simulink model "CAES_Expansion"  (R2022a)
settings: Solver=VariableStepAuto  StartTime=0.0  StopTime=100  RelTol=1e-3
values from neighbouring files (symbols this model uses):
  c1 = 1-c2    (= 0.95)    [CAES_Parameters.m]
  c2 = 0.05    [CAES_Parameters.m]
  Dt = 2    [CAES_Parameters.m]
  Fmax = 1.25+0.25    (= 1.5)    [CAES_Parameters.m]
  Fmin = 0    [CAES_Parameters.m]
  gmax = 1.25+0.25    (= 1.5)    [CAES_Parameters.m]
  gmin = 0.1    [CAES_Parameters.m]
  Ht = 3.9821    [CAES_Parameters.m]
  K4 = 0.8    [CAES_Parameters.m]
  K5 = 0.2    [CAES_Parameters.m]
  Kti = 2    [CAES_Parameters.m]
  KTi = 5    [CAES_Parameters.m]
  Ktp = 3    [CAES_Parameters.m]
  KTp = 7    [CAES_Parameters.m]
  R = 0.04    [CAES_Parameters.m]
  tau3 = 15    [CAES_Parameters.m]
  tau4 = 2.5    [CAES_Parameters.m]
  tauAV = 0.1    [CAES_Parameters.m]
  tauS = 0.05    [CAES_Parameters.m]
  tauSF = 0.4    [CAES_Parameters.m]
  tauTD = 0.3    [CAES_Parameters.m]
  tauTP = 0.02    [CAES_Parameters.m]
  Ts = 323.15    [CAES_Parameters.m]
  TxLPo = 668.15    [CAES_Parameters.m]
  Txref = 1    [CAES_Parameters.m]
  umax = 1.2+0.3    (= 1.5)    [CAES_Parameters.m]
  umin = 0    [CAES_Parameters.m]
libraries: slpidlib x2, spsGroundLib x2, spsLoadFlowBusLib x2, spsThreePhaseParallelRLCLoadLib x2, spsThreePhaseBreakerLib x1, spsSimplifiedSynchronousMachinepuUnitsLib x1, spspowerguiLib x1, spsVoltageMeasurementLib x1
settings Model: Creator=xiaojs20  LastModifiedBy=xiaojs20

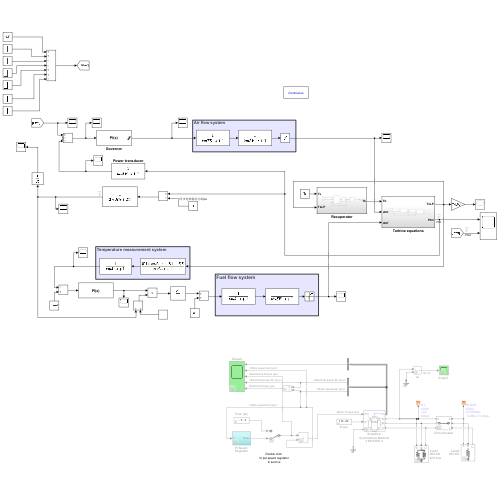
[thumbnail: Simulink's stored preview of the top-level diagram]
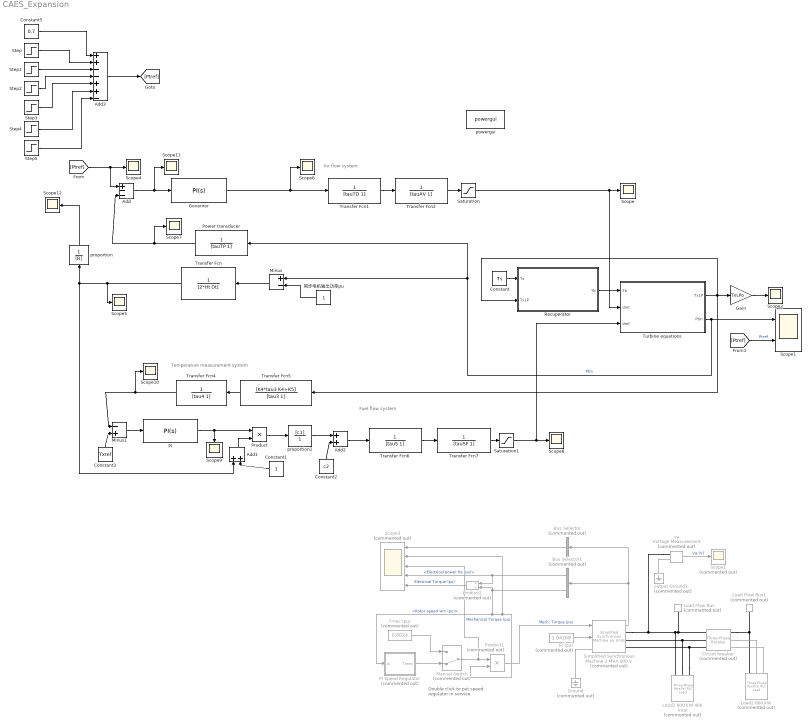
== system CAES_Expansion ==
  note: Fuel flow system
  note: Temperature measurement system
  note: Air flow system
  note: Double click
      | to put speed regulator
      | in service
  Add : Sum  Inputs=+--
  Add1 : Sum
  Add2 : Sum
  Add3 : Sum  Inputs=++--++-
  Bus Selector : BusSelector  Commented=on  OutputSignals=Stator current is_a (pu),Stator current is_b (pu),Stator current is_c (pu)  OutputAsBus=on
  Bus Selector1 : BusSelector  Commented=on  OutputSignals=Electrical power Pe (pu),Rotor speed wm (pu)
  Circuit breaker : spsThreePhaseBreakerLib/Three-Phase Breaker  Commented=on  InitialState=closed  SwitchA=on  SwitchB=on  SwitchC=on  SwitchTimes=[ 0.2 0.7*100 ]  External=off  BreakerResistance=1e-4  SnubberResistance=inf  SnubberCapacitance=0  Measurements=None
      settings: AttributesFormatString=\n
  Constant : Constant  Value=Ts
  Constant1 : Constant
  Constant2 : Constant  Value=c2
  Constant3 : Constant  Value=Txref
  Constant5 : Constant  Value=0.7
  Ei (pu) : Constant  Commented=on  Value=1.04268
  Gain : Gain  Gain=TxLPo
  Governor : slpidlib/PID Controller  Controller=PI  Form=Parallel  TimeDomain=Continuous-time  UseExternalTs=off  SampleTime=-1  IntegratorMethod=Forward Euler  FilterMethod=Forward Euler  ControllerParametersSource=internal  P=Ktp  I=Kti  UseKiTs=off  D=0  N=100  UseFilter=on  TunerSelectOption=Transfer Function Based (PID Tuner App)  InitialConditionSource=internal  InitialConditionForIntegrator=0  InitialConditionForFilter=0  DifferentiatorICPrevScaledInput=0  ExternalReset=none  TrackingMode=off  Kt=1  LimitOutput=on  SatLimitsSource=internal  UpperSaturationLimit=umax  LowerSaturationLimit=umin  LinearizeAsGain=on  AntiWindupMode=none  Kb=1  POutMin=[]  POutMax=[]  IOutMin=[]  IOutMax=[]  DOutMin=[]  DOutMax=[]  NOutMin=[]  NOutMax=[]  SumOutMin=[]  SumOutMax=[]  SaturationOutMin=[]  SaturationOutMax=[]  PParamMin=[]  PParamMax=[]  IParamMin=[]  IParamMax=[]  DParamMin=[]  DParamMax=[]  NParamMin=[]  NParamMax=[]  KbParamMin=[]  KbParamMax=[]  KtParamMin=[]  KtParamMax=[]  KbOutMin=[]  KbOutMax=[]  KtOutMin=[]  KtOutMax=[]  IntegratorOutMin=[]  IntegratorOutMax=[]  FilterOutMin=[]  FilterOutMax=[]  SumI1OutMin=[]  SumI1OutMax=[]  SumI2OutMin=[]  SumI2OutMax=[]  SumI3OutMin=[]  SumI3OutMax=[]  SumI4OutMin=[]  SumI4OutMax=[]  SumDOutMin=[]  SumDOutMax=[]  DifferentiatorOutMin=[]  DifferentiatorOutMax=[]  FilterDiffOutCoefMin=[]  FilterDiffOutCoefMax=[]  ReciprocalOutMin=[]  ReciprocalOutMax=[]  SumDenOutMin=[]  SumDenOutMax=[]  SumNumOutMin=[]  SumNumOutMax=[]  DivideOutMin=[]  DivideOutMax=[]  UdiffTsProdOutMin=[]  UdiffTsProdOutMax=[]  NTsProdOutMin=[]  NTsProdOutMax=[]  UintegralTsProdOutMin=[]  UintegralTsProdOutMax=[]  UngainTsProdOutMin=[]  UngainTsProdOutMax=[]  IntegratorContinuousStateAttributes=''  IntegratorStateMustResolveToSignalObject=off  IntegratorRTWStateStorageClass=Auto  FilterContinuousStateAttributes=''  FilterStateMustResolveToSignalObject=off  FilterRTWStateStorageClass=Auto  ParallelPVariant=InternalParameters  IdealPVariant=Disabled  IVariant=InternalParameters  DVariant=Disabled  IntegratorVariant=Continuous  SatVariant=Enabled  AWVariant=Passthrough  PCopyVariant=Disabled  TRVariant=Disabled  FdbkBlocksVariant=Forward  IdealPFdbkVariant=Disabled  SatFdbkVariant=Disabled  DerivativeFilterVariant=Disabled  NVariant=Disabled  NCopyVariant=Disabled_SignalSpec  FilterICVariant=Disabled  IntegratorICVariant=InternalICs  ExternalResetVariant=Disabled  TRSumVariant=Passthrough  SumFdbkVariant=Disabled  SumVariant=Sum_PI  TsampFilterVariant=InternalTs  TsampNgainVariant=Passthrough  TsampIntegralVariant=Passthrough  ExternalSaturationOutDataTypeStr=Inherit: Same as second input  aMode=0
  Ground : spsGroundLib/Ground  Commented=on  LConnTagsString=a
  Load Flow Bus : spsLoadFlowBusLib/Load Flow Bus  Commented=on  LConnTagsString=a  Phases=single  Connectors=on one side  ID=B1  Vbase=600  Vref=1  Vangle=0  VLF=1  VLFb=1  VLFc=1  angleLF=0  angleLFb=0  angleLFc=0
      settings: AttributesFormatString=%<ID>\n%<Vbase>V\n%<VLF>pu\n%<angleLF>deg.  SourceProductBaseCode=PS
  Load Flow Bus1 : spsLoadFlowBusLib/Load Flow Bus  Commented=on  LConnTagsString=a  Phases=single  Connectors=on one side  ID=BLOAD  Vbase=600  Vref=1  Vangle=0  VLF=0.9998  VLFb=1  VLFc=1  angleLF=-9.68e-011  angleLFb=0  angleLFc=0
      settings: AttributesFormatString=%<ID>\n%<Vbase>V\n%<VLF>pu\n%<angleLF>deg.  SourceProductBaseCode=PS
  Load1 800 kW 400 kvar : spsThreePhaseParallelRLCLoadLib/Three-Phase Parallel RLC Load  Commented=on  LConnTagsString=A|B|C  Configuration=Y (grounded)  NominalVoltage=600  Vabc=[1e3 1e3 1e3]  Vabcp=[1e3 1e3 1e3]  NominalFrequency=60  UnbalancedPower=off  ActivePower=800000  InductivePower=400e3  CapacitivePower=0  Pabc=[10e3 9e3 11e3]  QLabc=[100 90 110]  QCabc=[100 90 110]  Pabcp=[10e3 9e3 11e3]  QLabcp=[100 90 110]  QCabcp=[100 90 110]  Measurements=None  LoadType=constant Z
  Load2 800 kW : spsThreePhaseParallelRLCLoadLib/Three-Phase Parallel RLC Load  Commented=on  LConnTagsString=A|B|C  Configuration=Y (grounded)  NominalVoltage=600  Vabc=[1e3 1e3 1e3]  Vabcp=[1e3 1e3 1e3]  NominalFrequency=60  UnbalancedPower=off  ActivePower=800000  InductivePower=0  CapacitivePower=0  Pabc=[10e3 9e3 11e3]  QLabc=[100 90 110]  QCabc=[100 90 110]  Pabcp=[10e3 9e3 11e3]  QLabcp=[100 90 110]  QCabcp=[100 90 110]  Measurements=None  LoadType=constant Z
  Manual Switch : ManualSwitch  Commented=on  CurrentSetting=0
  Minus : Sum  Inputs=+-
  Minus1 : Sum  Inputs=-+
  PI : slpidlib/PID Controller  Controller=PI  Form=Parallel  TimeDomain=Continuous-time  UseExternalTs=off  SampleTime=-1  IntegratorMethod=Forward Euler  FilterMethod=Forward Euler  ControllerParametersSource=internal  P=KTp  I=KTi  UseKiTs=off  D=0  N=100  UseFilter=on  TunerSelectOption=Transfer Function Based (PID Tuner App)  InitialConditionSource=internal  InitialConditionForIntegrator=0  InitialConditionForFilter=0  DifferentiatorICPrevScaledInput=0  ExternalReset=none  TrackingMode=off  Kt=1  LimitOutput=off  SatLimitsSource=internal  UpperSaturationLimit=umax  LowerSaturationLimit=umin  LinearizeAsGain=on  AntiWindupMode=none  Kb=1  POutMin=[]  POutMax=[]  IOutMin=[]  IOutMax=[]  DOutMin=[]  DOutMax=[]  NOutMin=[]  NOutMax=[]  SumOutMin=[]  SumOutMax=[]  SaturationOutMin=[]  SaturationOutMax=[]  PParamMin=[]  PParamMax=[]  IParamMin=[]  IParamMax=[]  DParamMin=[]  DParamMax=[]  NParamMin=[]  NParamMax=[]  KbParamMin=[]  KbParamMax=[]  KtParamMin=[]  KtParamMax=[]  KbOutMin=[]  KbOutMax=[]  KtOutMin=[]  KtOutMax=[]  IntegratorOutMin=[]  IntegratorOutMax=[]  FilterOutMin=[]  FilterOutMax=[]  SumI1OutMin=[]  SumI1OutMax=[]  SumI2OutMin=[]  SumI2OutMax=[]  SumI3OutMin=[]  SumI3OutMax=[]  SumI4OutMin=[]  SumI4OutMax=[]  SumDOutMin=[]  SumDOutMax=[]  DifferentiatorOutMin=[]  DifferentiatorOutMax=[]  FilterDiffOutCoefMin=[]  FilterDiffOutCoefMax=[]  ReciprocalOutMin=[]  ReciprocalOutMax=[]  SumDenOutMin=[]  SumDenOutMax=[]  SumNumOutMin=[]  SumNumOutMax=[]  DivideOutMin=[]  DivideOutMax=[]  UdiffTsProdOutMin=[]  UdiffTsProdOutMax=[]  NTsProdOutMin=[]  NTsProdOutMax=[]  UintegralTsProdOutMin=[]  UintegralTsProdOutMax=[]  UngainTsProdOutMin=[]  UngainTsProdOutMax=[]  IntegratorContinuousStateAttributes=''  IntegratorStateMustResolveToSignalObject=off  IntegratorRTWStateStorageClass=Auto  FilterContinuousStateAttributes=''  FilterStateMustResolveToSignalObject=off  FilterRTWStateStorageClass=Auto  ParallelPVariant=InternalParameters  IdealPVariant=Disabled  IVariant=InternalParameters  DVariant=Disabled  IntegratorVariant=Continuous  SatVariant=Disabled  AWVariant=Passthrough  PCopyVariant=Disabled  TRVariant=Disabled  FdbkBlocksVariant=Forward  IdealPFdbkVariant=Disabled  SatFdbkVariant=Disabled  DerivativeFilterVariant=Disabled  NVariant=Disabled  NCopyVariant=Disabled_SignalSpec  FilterICVariant=Disabled  IntegratorICVariant=InternalICs  ExternalResetVariant=Disabled  TRSumVariant=Passthrough  SumFdbkVariant=Disabled  SumVariant=Sum_PI  TsampFilterVariant=InternalTs  TsampNgainVariant=Passthrough  TsampIntegralVariant=Passthrough  ExternalSaturationOutDataTypeStr=Inherit: Same as second input  aMode=0
  PI Speed Regulator : Subsystem  Commented=on
  Power transducer : TransferFcn  Denominator=[tauTP 1]
  Product : Product
  Product1 : Product  Commented=on  InputSameDT=on  SaturateOnIntegerOverflow=on  OutDataTypeStr=Inherit: Same as first input
  Product2 : Product  Commented=on  Inputs=*/  InputSameDT=on  SaturateOnIntegerOverflow=on  OutDataTypeStr=Inherit: Same as first input
  Recuperator : Subsystem
  Saturation : Saturate  UpperLimit=gmax  LowerLimit=gmin
  Saturation1 : Saturate  UpperLimit=Fmax  LowerLimit=Fmin  ZeroCross=off
  Scope{,2,4..12} (11 alike) : Scope
  Scope1 : Scope  NumInputPorts=2
  "Scope1 " : Scope  Commented=on
  Scope3 : Scope  Commented=on  NumInputPorts=5
  Simplified Synchronous Machine 2 MVA 600 V : spsSimplifiedSynchronousMachinepuUnitsLib/Simplified Synchronous Machine pu Units  Commented=on  ConnectionType=4-wire Y  MechanicalLoad=Mechanical power Pm  MeasurementBus=off  NominalParameters="[  2000e3, 600, 60 ]"  Mechanical=[ 0.6 , 0.0, 2 ]  InternalRL="[ 0.0036  0.16 ]"  InitialConditions=[0 7.01083 0.824535 0.824535 0.824535 -14.0377 -134.038 105.962 ]  IterativeDiscreteModel=Trapezoidal non iterative  TsBlock=-1  TsPowergui=0  LoadFlowParameters=[2 0 0 0]  Units=0  BusType=swing  Pref=0  Qref=0  Qmin=-Inf  Qmax=Inf  PLF=0  QLF=0
      settings: AttributesFormatString=\n  SourceProductBaseCode=PS
  Step : Step  Time=5  After=0.3  SampleTime=0  ZeroCross=off
  Step1 : Step  Time=20  After=0.3  SampleTime=0  ZeroCross=off
  Step2 : Step  Time=35  After=0.1  SampleTime=0  ZeroCross=off
  Step3 : Step  Time=50  After=0.1  SampleTime=0  ZeroCross=off
  Step4 : Step  Time=65  After=0.5  SampleTime=0  ZeroCross=off
  Step5 : Step  Time=80  After=0.5  SampleTime=0  ZeroCross=off
  Tmec (pu) : Constant  Commented=on  Value=0.8024
  Transfer Fcn : TransferFcn  Denominator=[2*Ht Dt]
  Transfer Fcn1 : TransferFcn  Denominator=[tauTD 1]
  Transfer Fcn2 : TransferFcn  Denominator=[tauAV 1]
  Transfer Fcn4 : TransferFcn  Denominator=[tau4 1]
  Transfer Fcn5 : TransferFcn  Numerator=[K4*tau3 K4+K5]  Denominator=[tau3 1]
  Transfer Fcn6 : TransferFcn  Denominator=[tauS 1]
  Transfer Fcn7 : TransferFcn  Denominator=[tauSF 1]
  Turbine equations : Subsystem
  output Ground1 : spsGroundLib/Ground  Commented=on  LConnTagsString=a
  powergui : spspowerguiLib/powergui  Priority=1  SimulationMode=Continuous  SampleTime=50e-6  frequency=60  Iterations=50  frequencyindice=60  Pbase=100e6  ErrMax=1e-4  UnitsV=kV  UnitsW=MW  buscounter=0  FunctionMessages=off  echomessages=off  EnableUseOfTLC=off  CurrentSourceSwitches=off  DisableSnubberDevices=off  DisableRonSwitches=off  DisableVfSwitches=off  DisplayEquations=off  AutomaticDiscreteSolvers=off  SolverType=Tustin/Backward Euler (TBE)  Interpol=off  ExternalGateDelay=off  methode=off  Ts=100  x0status=blocks  SPID=on  SwTol=0  HookPort=off  NonlinearTolerance=1e-4  nMaxIteration=100  ContinueOnMaxIteration=off  RestoreLinks=warning  ResistiveCurrentMeasurement=off  Frange=[0:2:500]  Ylog=off  Xlog=on  ShowGrid=off  save=off  variable=ZData  structure=0  ZoomFFT=off  StartTime=0.0  cycles=1  DisplayStyle=1  fundamental=60  FreqAxis=off  MaxFrequency=1000  frequencyindicesteady=1  RmsSteady=1  display=off
  proportion : TransferFcn  Denominator=[R]
  proportion1 : TransferFcn  Numerator=[c1]  Denominator=[1]
  va : spsVoltageMeasurementLib/Voltage Measurement  Tag=PoWeRsYsTeMmEaSuReMeNt  Commented=on  PhasorSimulation=off  OutputType=Magnitude  PSBequivalent=0
  同步电机输出功率pu : Constant
  wires:
  Transfer Fcn/1 -> Scope5/1, Add1/1, proportion/1
  Minus/1 -> Transfer Fcn/1
  Turbine equations/2(Ptm) -> Power transducer/1, Minus/1, Scope1/1  "Ptm"
  Governor/1 -> Scope6/1, Transfer Fcn1/1
  Transfer Fcn1/1 -> Transfer Fcn2/1
  Transfer Fcn2/1 -> Saturation/1
  Add/1 -> Scope11/1, Governor/1
  Power transducer/1 -> Scope7/1, Add/3
  Turbine equations/1(TxLP) -> Gain/1, Transfer Fcn5/1, Recuperator/2(TxLP)
  Transfer Fcn5/1 -> Transfer Fcn4/1
  Transfer Fcn4/1 -> Scope10/1, Minus1/1
  Minus1/1 -> PI/1
  Constant3/1 -> Minus1/2
  PI/1 -> Product/1, Scope9/1
  Constant1/1 -> Add1/2
  Add1/1 -> Product/2
  Product/1 -> proportion1/1
  proportion1/1 -> Add2/1
  Constant2/1 -> Add2/2
  Add2/1 -> Transfer Fcn6/1
  Transfer Fcn6/1 -> Transfer Fcn7/1
  Transfer Fcn7/1 -> Saturation1/1
  Recuperator/1(Tb) -> Turbine equations/1(Tb)
  Saturation/1 -> Scope/1, Turbine equations/2(dmt)
  Saturation1/1 -> Scope8/1, Turbine equations/3(dmf)
  Constant/1 -> Recuperator/1(Ts)
  Add3/1 -> [Ptref]
  Step/1 -> Add3/2
  Constant5/1 -> Add3/1
  Step1/1 -> Add3/3
  Step2/1 -> Add3/4
  Step3/1 -> Add3/5
  Step4/1 -> Add3/6
  Step5/1 -> Add3/7
  [Ptref] -> Add/1, Scope4/1
  Bus Selector1/1 -> Product2/1, Scope3/4  "<Electrical power Pe (pu)>"
  Simplified Synchronous Machine 2 MVA 600 V/1 -> Bus Selector1/1, Bus Selector/1
  Bus Selector1/2 -> PI Speed Regulator/1(w), Scope3/2, Product1/2, Product2/2  "<Rotor speed wm (pu)>"
  Product1/1 -> Simplified Synchronous Machine 2 MVA 600 V/1  "Mech. Torque (pu)"
  Bus Selector/1 -> Scope3/1
  Product2/1 -> Scope3/5  "Electrical Torque (pu)"
  Manual Switch/1 -> Product1/1, Scope3/3  "Mechanical Torque (pu)"
  Ei (pu)/1 -> Simplified Synchronous Machine 2 MVA 600 V/2
  va/1 -> "Scope1 "/1  "Va (V)"
  PI Speed Regulator/1(Tmec) -> Manual Switch/2
  Tmec (pu)/1 -> Manual Switch/1
  [Ptref] -> Scope1/2  "Ptref"
  proportion/1 -> Scope12/1
  Gain/1 -> Scope2/1
  同步电机输出功率pu/1 -> Minus/2
  connections:
  va/LConn1 -- Circuit breaker/LConn1 -- Load Flow Bus/LConn1 -- Load1 800 kW 400 kvar/LConn1 -- Simplified Synchronous Machine 2 MVA 600 V/RConn1
  Load1 800 kW 400 kvar/LConn2 -- Circuit breaker/LConn2 -- Simplified Synchronous Machine 2 MVA 600 V/RConn2
  Load Flow Bus1/LConn1 -- Circuit breaker/RConn1 -- Load2 800 kW/LConn1
  Load1 800 kW 400 kvar/LConn3 -- Circuit breaker/LConn3 -- Simplified Synchronous Machine 2 MVA 600 V/RConn3
  output Ground1/LConn1 -- va/LConn2
  Simplified Synchronous Machine 2 MVA 600 V/LConn1 -- Ground/LConn1
  Circuit breaker/RConn2 -- Load2 800 kW/LConn2
  Circuit breaker/RConn3 -- Load2 800 kW/LConn3

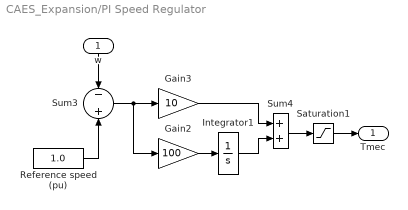
== system CAES_Expansion/PI Speed Regulator ==
  w : Inport
  Gain2 : Gain  Gain=100  SaturateOnIntegerOverflow=on  OutDataTypeStr=Inherit: Same as input  ParamDataTypeStr=Inherit: Same as input
  Gain3 : Gain  Gain=10  SaturateOnIntegerOverflow=on  OutDataTypeStr=Inherit: Same as input  ParamDataTypeStr=Inherit: Same as input
  Integrator1 : Integrator  InitialCondition=0.8024  LimitOutput=on  UpperSaturationLimit=1  LowerSaturationLimit=0  ZeroCross=off
  Reference speed (pu) : Constant  Value=1.0
  Saturation1 : Saturate  UpperLimit=1  LowerLimit=0  ZeroCross=off
  Sum3 : Sum  Inputs=-+  InputSameDT=on  SaturateOnIntegerOverflow=on  OutDataTypeStr=Inherit: Same as first input
  Sum4 : Sum  InputSameDT=on  SaturateOnIntegerOverflow=on  OutDataTypeStr=Inherit: Same as first input
  Tmec : Outport  VectorParamsAs1DForOutWhenUnconnected=off
  wires:
  Gain3/1 -> Sum4/1
  Gain2/1 -> Integrator1/1
  Sum3/1 -> Gain3/1, Gain2/1
  Integrator1/1 -> Sum4/2
  Reference speed (pu)/1 -> Sum3/2
  Sum4/1 -> Saturation1/1
  w/1 -> Sum3/1
  Saturation1/1 -> Tmec/1

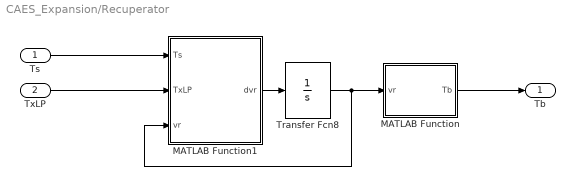
== system CAES_Expansion/Recuperator ==
  Ts : Inport
  TxLP : Inport  Port=2
  MATLAB Function : MATLAB Function  TreatAsAtomicUnit=on
  MATLAB Function1 : MATLAB Function  TreatAsAtomicUnit=on
  Transfer Fcn8 : TransferFcn  Denominator=[1 0]
  Tb : Outport
  wires:
  MATLAB Function1/1(dvr) -> Transfer Fcn8/1
  TxLP/1 -> MATLAB Function1/2(TxLP)
  Transfer Fcn8/1 -> MATLAB Function/1(vr), MATLAB Function1/3(vr)
  MATLAB Function/1(Tb) -> Tb/1
  Ts/1 -> MATLAB Function1/1(Ts)

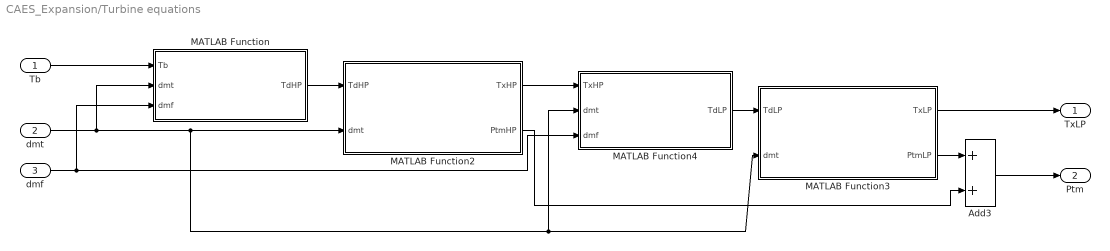
== system CAES_Expansion/Turbine equations ==
  Tb : Inport
  dmt : Inport  Port=2
  dmf : Inport  Port=3
  Add3 : Sum
  MATLAB Function : MATLAB Function  TreatAsAtomicUnit=on
  MATLAB Function2 : MATLAB Function  TreatAsAtomicUnit=on
  MATLAB Function3 : MATLAB Function  TreatAsAtomicUnit=on
  MATLAB Function4 : MATLAB Function  TreatAsAtomicUnit=on
  TxLP : Outport
  Ptm : Outport  Port=2
  wires:
  MATLAB Function2/2(PtmHP) -> Add3/2
  Add3/1 -> Ptm/1
  dmf/1 -> MATLAB Function4/3(dmf), MATLAB Function/3(dmf)
  dmt/1 -> MATLAB Function/2(dmt), MATLAB Function4/2(dmt), MATLAB Function3/2(dmt), MATLAB Function2/2(dmt)
  MATLAB Function/1(TdHP) -> MATLAB Function2/1(TdHP)
  Tb/1 -> MATLAB Function/1(Tb)
  MATLAB Function3/2(PtmLP) -> Add3/1
  MATLAB Function3/1(TxLP) -> TxLP/1
  MATLAB Function4/1(TdLP) -> MATLAB Function3/1(TdLP)
  MATLAB Function2/1(TxHP) -> MATLAB Function4/1(TxHP)

== matlab function CAES_Expansion/Recuperator/MATLAB Function1 ==
  data: dvr output; Ts input; TxLP input; vr input
function dvr=dvr_solver(Ts,TxLP,vr)
    TxLPo=668.15;
    Tbo=599.15;
    eps_r=0.80;
    tauR=25;

    dvr=(1/tauR)*(eps_r*(TxLP*TxLPo-Ts)/(Tbo)-vr);
end

== matlab function CAES_Expansion/Recuperator/MATLAB Function ==
  data: Tb output; vr input
function Tb=Tb_solver(vr)
    Ts=323.15;
    Tbo=599.15;
    Tb=Ts/Tbo+vr;
end

== matlab function CAES_Expansion/Turbine equations/MATLAB Function ==
  data: Tb input; TdHP output; dmt input; dmf input
function TdHP=HPburner_solver(Tb,dmt,dmf)
    Tbo=599.15;
    TdHPo=823.15; 

    TdHP=Tb*(Tbo/TdHPo)+((TdHPo-Tbo)/TdHPo)*(dmf/dmt);
end

== matlab function CAES_Expansion/Turbine equations/MATLAB Function2 ==
  data: TdHP input; dmt input; TxHP output; PtmHP output
function [TxHP,PtmHP]=HPexpander_solver(TdHP,dmt)
    TdHPo=823.15; 
    TxHPo=612.15;
    gamma=1.4;
    g=(gamma-1)/gamma;
    pi_tHPo=3.818;
    eta_tHPi=0.8065;
    cp=1.055;
    Ptmo=280;
    dmto=417;

    TxHP=(TdHPo*TdHP)/TxHPo*(1-(1-1/(pi_tHPo*dmt)^g)*eta_tHPi);
    PtmHP=(eta_tHPi*cp*dmto)/(1e3*Ptmo)*dmt*(TdHPo*TdHP-TxHPo*TxHP);

end

== matlab function CAES_Expansion/Turbine equations/MATLAB Function3 ==
  data: TdLP input; dmt input; TxLP output; PtmLP output
function [TxLP,PtmLP]=LPexpander_solver(TdLP,dmt)
    TdHPo=823.15; TdLPo=1098.2; TxHPo=612.15; TxLPo=668.15;
    gamma=1.4;
    g=(gamma-1)/gamma;
    pi_tHPo=3.818; pi_tLPo=10.856;
    eta_tHPi=0.8065; eta_tLPi=0.7926;
    cp=1.055;
    Ptmo=280;
    dmto=417;

    TxLP=(TdLPo*TdLP)/TxLPo*(1-(1-1/(pi_tLPo*dmt)^g)*eta_tLPi);
    PtmLP=(eta_tLPi*cp*dmto)/(1e3*Ptmo)*dmt*(TdLPo*TdLP-TxLPo*TxLP);

end

== matlab function CAES_Expansion/Turbine equations/MATLAB Function4 ==
  data: TxHP input; TdLP output; dmt input; dmf input
function TdLP=LPburner_solver(TxHP,dmt,dmf)
    Tbo=599.15;
    TdHPo=823.15; TdLPo=1098.2; TxHPo=612.15; TxLPo=668.15;
    TdLP=TxHP*(TxHPo/TdLPo)+((TdLPo-TxHPo)/TdLPo)*(dmf/dmt);
end
